simulink model "perbandingan_3TFlevel"  (R2021b)
settings: Solver=VariableStepAuto  StartTime=0.0  StopTime=750  RelTol=1e-3
settings Model: Creator=Asus  LastModifiedBy=Asus

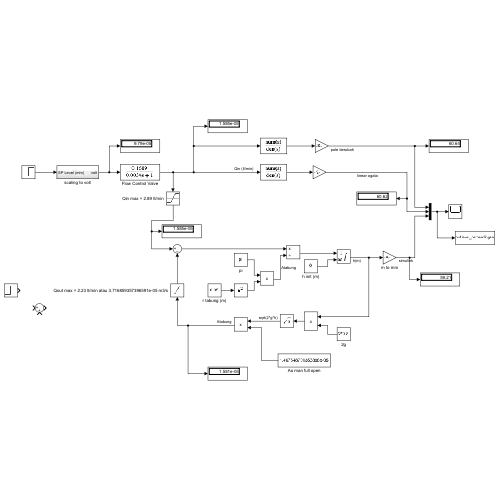
[thumbnail: Simulink's stored preview of the top-level diagram]
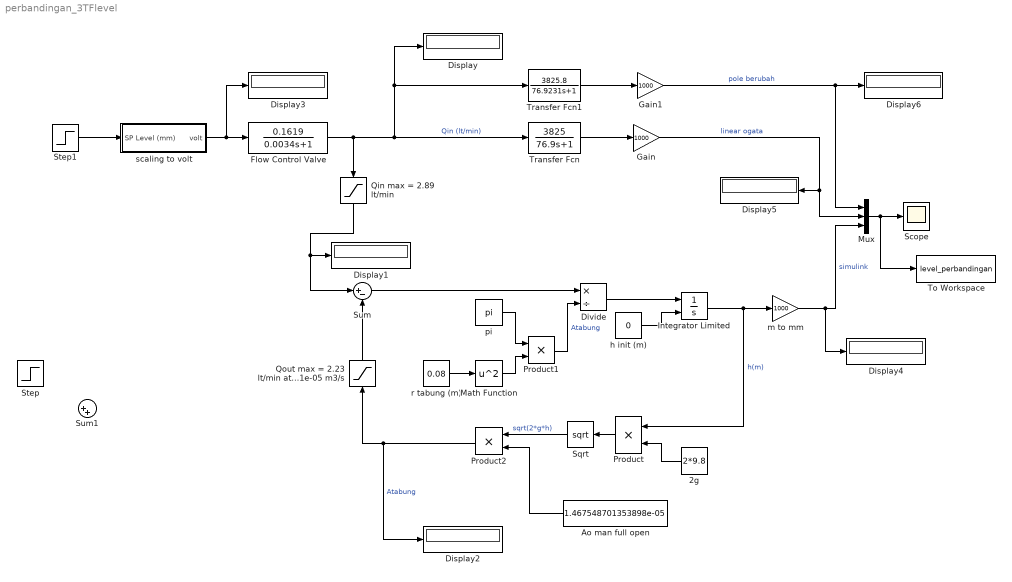
== system perbandingan_3TFlevel ==
  2g : Constant  Value=2*9.8
  Ao man full open : Constant  Value=1.467548701353898e-05
  Display{,1..6} (7 alike) : Display
  Divide : Product  Inputs=*/
  Flow Control Valve : TransferFcn  Numerator=[0.1619]  Denominator=[0.0034 1]
  Gain : Gain  Gain=1000
  Gain1 : Gain  Gain=1000
  Integrator Limited : Integrator  InitialConditionSource=external  LimitOutput=on  UpperSaturationLimit=1  LowerSaturationLimit=0
  Math Function : Math  Operator=square  SaturateOnIntegerOverflow=on
  Mux : Mux  Inputs=3
  Product : Product
  Product1 : Product
  Product2 : Product
  Qin max = 2.89 lt/min : Saturate  UpperLimit=2.89254556517870  LowerLimit=0
  Qout max = 2.23 lt/min atau 3.716859357396591e-05 m3/s : Saturate  UpperLimit=3.716859357396591e-05  LowerLimit=0
  Scope : Scope
  Sqrt : Sqrt  SaturateOnIntegerOverflow=on
  Step : Step  Time=0  After=9.9640e-05  SampleTime=0
  Step1 : Step  Time=0  After=42.1797  SampleTime=0
  Sum : Sum  Inputs=|+-
  Sum1 : Sum  Inputs=|++
  To Workspace : ToWorkspace  VariableName=level_perbandingan  SampleTime=-1
  Transfer Fcn : TransferFcn  Numerator=[3825]  Denominator=[76.9 1]
  Transfer Fcn1 : TransferFcn  Numerator=[3825.8]  Denominator=[76.9231 1]
  h init (m) : Constant  Value=0
  m to mm : Gain  Gain=1000
  pi : Constant  Value=pi
  r tabung (m) : Constant  Value=0.08
  scaling to volt : Subsystem
  wires:
  Transfer Fcn/1 -> Gain/1
  Gain/1 -> Mux/2, Display5/1  "linear ogata"
  pi/1 -> Product1/1
  Product/1 -> Sqrt/1
  h init (m)/1 -> Integrator Limited/2
  Integrator Limited/1 -> Product/1, m to mm/1  "h(m)"
  Math Function/1 -> Product1/2
  r tabung (m)/1 -> Math Function/1
  2g/1 -> Product/2
  Divide/1 -> Integrator Limited/1
  Sum/1 -> Divide/1
  Product1/1 -> Divide/2  "Atabung"
  m to mm/1 -> Display4/1, Mux/3  "simulink"
  Mux/1 -> To Workspace/1, Scope/1
  Sqrt/1 -> Product2/1  "sqrt(2*g*h)"
  Ao man full open/1 -> Product2/2
  Product2/1 -> Display2/1, Qout max = 2.23 lt/min atau 3.716859357396591e-05 m3/s/1  "Atabung"
  Qout max = 2.23 lt/min atau 3.716859357396591e-05 m3/s/1 -> Sum/2
  scaling to volt/1(volt) -> Display3/1, Flow Control Valve/1
  Qin max = 2.89 lt/min/1 -> Sum/1, Display1/1
  Step1/1 -> scaling to volt/1(SP Level (mm))
  Flow Control Valve/1 -> Display/1, Transfer Fcn1/1, Transfer Fcn/1, Qin max = 2.89 lt/min/1  "Qin (lt/min)"
  Transfer Fcn1/1 -> Gain1/1
  Gain1/1 -> Mux/1, Display6/1  "pole berubah"

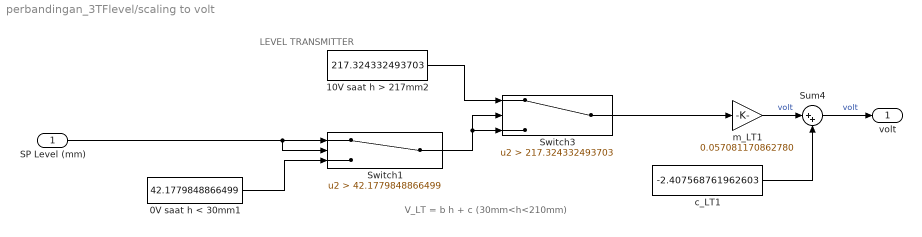
== system perbandingan_3TFlevel/scaling to volt ==
  note: LEVEL TRANSMITTER
  note: V_LT = b h + c (30mm<h<210mm)
  SP Level (mm) : Inport
  0V saat h < 30mm1 : Constant  Value=42.1779848866499
  10V saat h > 217mm2 : Constant  Value=217.324332493703
  Sum4 : Sum  Inputs=|++
  Switch1 : Switch  Criteria=u2 > Threshold  Threshold=42.1779848866499
  Switch3 : Switch  Criteria=u2 > Threshold  Threshold=217.324332493703
  c_LT1 : Constant  Value=-2.407568761962603
  m_LT1 : Gain  Gain=0.057081170862780
  volt : Outport
  wires:
  Switch1/1 -> Switch3/2, Switch3/3
  SP Level (mm)/1 -> Switch1/1, Switch1/2
  10V saat h > 217mm2/1 -> Switch3/1
  0V saat h < 30mm1/1 -> Switch1/3
  m_LT1/1 -> Sum4/1  "volt"
  Switch3/1 -> m_LT1/1
  c_LT1/1 -> Sum4/2
  Sum4/1 -> volt/1  "volt"
